simulink model "TSMC_MPC_PMSM"  (R2016b)
settings: Solver=ode23tb  StartTime=0.0  StopTime=0.6  RelTol=1e-4
InitFcn:
  | Ts=10e-6;
  | Rs=0.958;
  | Rf=0.2;
  | Lf=0.002;
  | Cf=0.000021;
  | L=0.000395;
  | Pn=4;
  | flux=0.1827;
  | frq=50;
  | Ld=0.000395;
  | Lq=0.000395;
  | R=0.958;
undefined symbols (not defined in the file or in its folder): DiscIntNeverNeededParam
libraries: powerlib x56, powerlib_extras x2
settings Model: Creator=ChenNingke  LastModifiedBy=CNK
settings SolverCC: MaxConsecutiveZCs=100000  ZeroCrossAlgorithm=Adaptive
settings DebuggingCC: MaskedZcDiagnostic=none

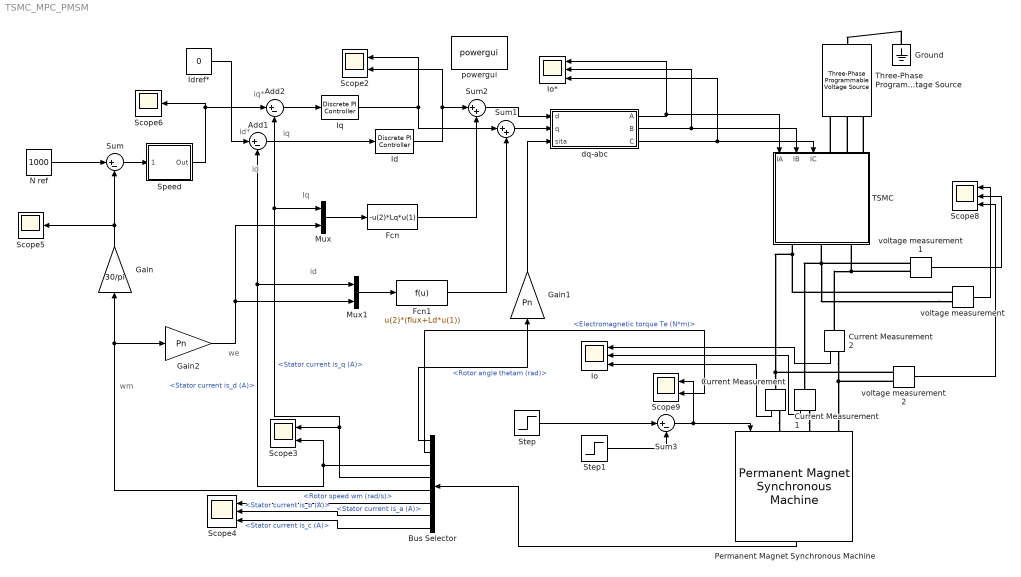
== system TSMC_MPC_PMSM ==
  note: we
  note: wm
  note: iq
  note: id
  note: id*
  note: iq*
  note: id
  note: Iq
  Add1 : Sum  Inputs=|+-
  Add2 : Sum  Inputs=|+-
  Bus Selector : BusSelector  OutputSignals=Rotor angle thetam (rad),Electromagnetic torque Te (N*m),Stator current is_d (A),Stator current is_q (A),Rotor speed wm (rad/s),Stator current is_a (A),Stator current is_b (A),Stator current is_c (A)
  Current Measurement : powerlib/Measurements/Current Measurement  PhasorSimulation=off  OutputType=Complex  PSBequivalent=0
  Current Measurement1 : powerlib/Measurements/Current Measurement  PhasorSimulation=off  OutputType=Complex  PSBequivalent=0
  Current Measurement2 : powerlib/Measurements/Current Measurement  PhasorSimulation=off  OutputType=Complex  PSBequivalent=0
  Fcn : Fcn  Expr=-u(2)*Lq*u(1)
  Fcn1 : Fcn  Expr=u(2)*(flux+Ld*u(1))
  Gain : Gain  Gain=30/pi
  Gain1 : Gain  Gain=Pn
  Gain2 : Gain  Gain=Pn
  Ground : powerlib/Elements/Ground  LConnTagsString=a
  Id : powerlib_extras/Discrete  Control Blocks/Discrete PI Controller  Kp=Ld*1100  Ki=R*1100  Par_Limits=[311*0.9*sqrt(1/3) -311*0.9*sqrt(1/3)]  Init=0  Ts=Ts
  Idref* : Constant  Value=0
  Io : Scope  NumInputPorts=3
  Io* : Scope  NumInputPorts=3
  Iq : powerlib_extras/Discrete  Control Blocks/Discrete PI Controller  Kp=Lq*1100  Ki=R*1100  Par_Limits=[311*0.9*sqrt(1/3) -311*0.9*sqrt(1/3)]  Init=0  Ts=Ts
  Mux : Mux  Inputs=2
  Mux1 : Mux  Inputs=2
  "N ref " : Constant  Value=1000
  Permanent Magnet Synchronous Machine : powerlib/Machines/Permanent Magnet Synchronous Machine  NbPhases=3  FluxDistribution=Sinusoidal  RotorType=Round  MechanicalLoad=Torque Tm  PresetModel=No  ShowDetailedParameters=on  MeasurementBus=off  Resistance=0.958  Inductance=8.5e-3  dqInductances=[Ld,Lq]  La=0.000395  MachineConstant=Flux linkage established by magnets (V.s)  Flux=0.1827  VoltageCst=132.5525  TorqueCst=1.0962  Flat=120  Mechanical=[0.003 0 4 0]  PolePairs=4  InitialConditions=[0,0, 0,0]  InitialConditions5ph=[0 0 0 0 0 0]  TsPowergui=0  TsBlock=-1  RefAngle=90 degrees behind phase A axis (modified Park)
  Scope2 : Scope  NumInputPorts=2
  Scope3 : Scope  NumInputPorts=2
  Scope4 : Scope  NumInputPorts=3
  Scope5 : Scope
  Scope6 : Scope
  Scope8 : Scope  NumInputPorts=3
  Scope9 : Scope  NumInputPorts=2
  Speed : Subsystem  AncestorBlock=|  DialogController=POWERSYS.PowerSysDialog  mask(Discrete PI Controller){Kpw=0.14, Kiw=0.14*50, Ba=0.013, Par_Limits=[15 -15], Init=0, Ts=Ts}
      | powerlib_extras/Discrete 
      | Control Blocks/Discrete
      | PI Controller
      mask prompts: Kpw "Proportional gain (Kp):"; Kiw "Integral gain (Ki):"; Ba "feedback gain (Ba)"; Par_Limits "Output limits: [ Upper   Lower ]"; Init "Output initial value:"; Ts "Sample time:"
      mask help: This block implements a discrete PI controller.
      mask init:
      | UpperLimit=Par_Limits(1);
      | LowerLimit=Par_Limits(2);
      | power_initmask();
      mask Help: This block is part of a subset of blocks in the Extras library that does not have documentation associated with it, other than the block mask description.
      mask Display: disp('PI');
  Step : Step  Time=0.2  After=10  SampleTime=Ts
  Step1 : Step  Time=0.4  After=3  SampleTime=Ts
  Sum : Sum  Inputs=|+-
  Sum1 : Sum  Inputs=|++
  Sum2 : Sum  Inputs=|++
  Sum3 : Sum  Inputs=|+-
  TSMC : Subsystem
  Three-Phase Programmable Voltage Source : powerlib/Electrical Sources/Three-Phase Programmable Voltage Source  PositiveSequence=[220 0 60]  VariationEntity=None  VariationType=Table of time-amplitude pairs  VariationTypeAlt=Step  VariationStep=0.5  VariationRate=10  VariationMagnitude=0.3  VariationFrequency=2  VariationTiming=[1 2]  VariationPhaseA=off  Amplitudes=[1 0.8 1.2 1.0]  TimeValues=[0 0.1 0.15 0.2]  HarmonicGeneration=off  HarmonicA=[3 0.2 -25 0]  HarmonicB=[2 0.15 35 2]  Timing="[0.05  3]"  BusType=swing  Pref=0  Qref=0  Qmin=-inf  Qmax=inf
  dq-abc : Subsystem
  powergui : powerlib/powergui  Priority=1  SimulationMode=Continuous  SolverType=Tustin/Backward Euler (TBE)  SampleTime=50e-6  frequency=60  SPID=off  DisableSnubberDevices=off  DisableRonSwitches=off  DisableVfSwitches=off  SwTol=0  DisplayEquations=off  Interpol=off  ExternalGateDelay=off  methode=off  Ts=10  FunctionMessages=off  echomessages=off  HookPort=off  EnableUseOfTLC=off  x0status=blocks  frequencyindice=0  Pbase=100e6  ErrMax=1e-4  Iterations=50  UnitsV=kV  UnitsW=MW  buscounter=0  RestoreLinks=warning  ResistiveCurrentMeasurement=off  Frange=[0:2:500]  Ylog=off  Xlog=on  ShowGrid=off  save=off  variable=ZData  structure=Io  ZoomFFT=off  StartTime=0.0  cycles=1  DisplayStyle=1  fundamental=60  FreqAxis=off  MaxFrequency=1000  frequencyindicesteady=1  RmsSteady=1  display=off
  voltage measurement : powerlib/Measurements/Voltage Measurement  PhasorSimulation=off  OutputType=Complex  PSBequivalent=0
  voltage measurement1 : powerlib/Measurements/Voltage Measurement  PhasorSimulation=off  OutputType=Complex  PSBequivalent=0
  voltage measurement2 : powerlib/Measurements/Voltage Measurement  PhasorSimulation=off  OutputType=Complex  PSBequivalent=0
  wires:
  dq-abc/1("A ") -> TSMC/1(IA), Io*/1
  dq-abc/2("B ") -> TSMC/2(IB), Io*/2
  Permanent Magnet Synchronous Machine/1 -> Bus Selector/1
  Bus Selector/5 -> Gain2/1, Gain/1  "<Rotor speed wm (rad/s)>"
  "N ref "/1 -> Sum/1
  Speed/1(Out) -> Add2/1, Scope6/1
  Id/1 -> Scope2/2, Sum2/1
  Iq/1 -> Sum1/1, Scope2/1
  Idref*/1 -> Add1/1
  Bus Selector/3 -> Mux1/1, Add1/2, Scope3/2  "<Stator current is_d (A)>"
  Bus Selector/4 -> Scope3/1, Mux/1, Add2/2  "<Stator current is_q (A)>"
  dq-abc/3("C ") -> TSMC/3(IC), Io*/3
  Gain/1 -> Sum/2, Scope5/1
  Bus Selector/8 -> Scope4/3  "<Stator current is_c (A)>"
  Bus Selector/7 -> Scope4/2  "<Stator current is_b (A)>"
  Bus Selector/6 -> Scope4/1  "<Stator current is_a (A)>"
  Bus Selector/1 -> Gain1/1  "<Rotor angle thetam (rad)>"
  Sum/1 -> Speed/1(Error)
  Add2/1 -> Iq/1
  Add1/1 -> Id/1
  Sum2/1 -> dq-abc/1(d)
  Sum1/1 -> dq-abc/2(q)
  voltage measurement/1 -> Scope8/1
  voltage measurement1/1 -> Scope8/2
  voltage measurement2/1 -> Scope8/3
  Current Measurement/1 -> Io/3
  Current Measurement1/1 -> Io/2
  Current Measurement2/1 -> Io/1
  Gain1/1 -> dq-abc/3(sita)
  Mux/1 -> Fcn/1
  Mux1/1 -> Fcn1/1
  Gain2/1 -> Mux/2, Mux1/2
  Fcn/1 -> Sum2/2
  Fcn1/1 -> Sum1/2
  Step/1 -> Sum3/1
  Sum3/1 -> Permanent Magnet Synchronous Machine/1, Scope9/1
  Step1/1 -> Sum3/2
  Bus Selector/2 -> Scope9/2  "<Electromagnetic torque Te (N*m)>"
  connections:
  Current Measurement/LConn1 -- voltage measurement/LConn1 -- TSMC/RConn1 -- voltage measurement2/LConn1
  voltage measurement/LConn2 -- Current Measurement1/LConn1 -- TSMC/RConn2 -- voltage measurement1/LConn1
  Permanent Magnet Synchronous Machine/LConn3 -- Current Measurement2/RConn1 -- voltage measurement2/LConn2
  voltage measurement1/LConn2 -- Current Measurement2/LConn1 -- TSMC/RConn3
  TSMC/LConn3 -- Three-Phase Programmable Voltage Source/RConn3
  TSMC/LConn2 -- Three-Phase Programmable Voltage Source/RConn2
  Ground/LConn1 -- Three-Phase Programmable Voltage Source/LConn1
  TSMC/LConn1 -- Three-Phase Programmable Voltage Source/RConn1
  Current Measurement1/RConn1 -- Permanent Magnet Synchronous Machine/LConn2
  Current Measurement/RConn1 -- Permanent Magnet Synchronous Machine/LConn1

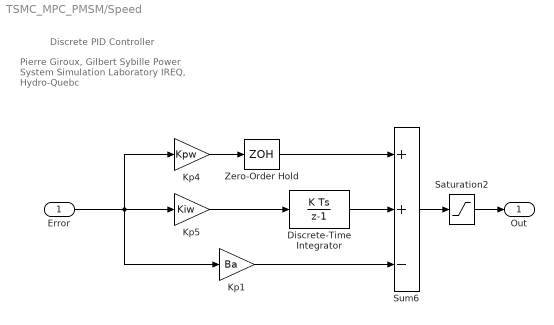
== system TSMC_MPC_PMSM/Speed ==
  note: Discrete PID Controller
  note: Pierre Giroux, Gilbert Sybille
      | Power System Simulation Laboratory
      | IREQ, Hydro-Quebc
  Error : Inport  SampleTime=Ts
  Discrete-Time Integrator : DiscreteIntegrator  InitialCondition=Init  SampleTime=Ts  LimitOutput=on  UpperSaturationLimit=UpperLimit  LowerSaturationLimit=LowerLimit  ICPrevOutput=DiscIntNeverNeededParam  ICPrevScaledInput=DiscIntNeverNeededParam
  Kp1 : Gain  Gain=Ba  SampleTime=Ts  SaturateOnIntegerOverflow=on  OutDataTypeStr=Inherit: Same as input  ParamDataTypeStr=Inherit: Same as input
  Kp4 : Gain  Gain=Kpw  SampleTime=Ts  SaturateOnIntegerOverflow=on  OutDataTypeStr=Inherit: Same as input  ParamDataTypeStr=Inherit: Same as input
  Kp5 : Gain  Gain=Kiw  SampleTime=Ts  SaturateOnIntegerOverflow=on  OutDataTypeStr=Inherit: Same as input  ParamDataTypeStr=Inherit: Same as input
  Saturation2 : Saturate  UpperLimit=UpperLimit  LowerLimit=LowerLimit  SampleTime=Ts
  Sum6 : Sum  Inputs=++-  SampleTime=Ts  SaturateOnIntegerOverflow=on  InputSameDT=on  OutDataTypeStr=Inherit: Same as first input
  Zero-Order Hold : ZeroOrderHold  SampleTime=Ts
  Out : Outport  SampleTime=Ts  InitialOutput=0
  wires:
  Error/1 -> Kp1/1, Kp5/1, Kp4/1
  Zero-Order Hold/1 -> Sum6/1
  Saturation2/1 -> Out/1
  Discrete-Time Integrator/1 -> Sum6/2
  Kp4/1 -> Zero-Order Hold/1
  Kp5/1 -> Discrete-Time Integrator/1
  Sum6/1 -> Saturation2/1
  Kp1/1 -> Sum6/3

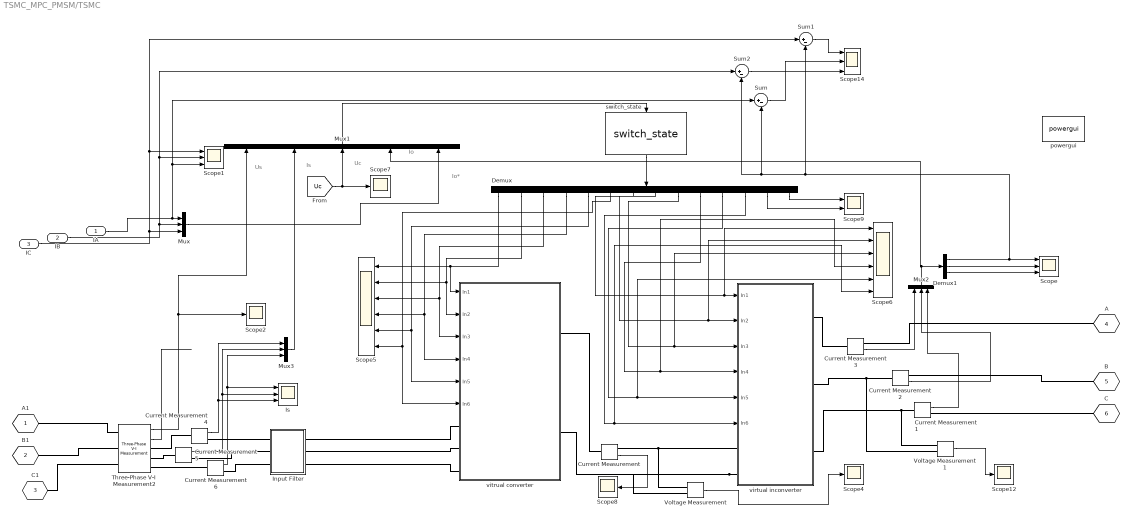
== system TSMC_MPC_PMSM/TSMC ==
  note: Us
  note: Is
  note: Io*
  note: Io
  note: Uc
  IA : Inport
  IB : Inport  Port=2
  IC : Inport  Port=3
  Current Measurement{,1..6} (7 alike) : powerlib/Measurements/Current Measurement  PhasorSimulation=off  OutputType=Complex  PSBequivalent=0
  Demux : Demux  Outputs=14
  Demux1 : Demux  Outputs=3
  Input Filter : Subsystem
  Is : Scope  NumInputPorts=3
  Mux : Mux  Inputs=3
  Mux1 : Mux  Inputs=5
  Mux2 : Mux  Inputs=3
  Mux3 : Mux  Inputs=3
  Scope : Scope  NumInputPorts=3
  Scope1 : Scope  NumInputPorts=3
  Scope{2,4,7..8,12} (5 alike) : Scope
  Scope14 : Scope  NumInputPorts=3
  Scope5 : Scope  NumInputPorts=6
  Scope6 : Scope  NumInputPorts=6
  Scope9 : Scope  NumInputPorts=2
  Sum : Sum  Inputs=|+-
  Sum1 : Sum  Inputs=|+-
  Sum2 : Sum  Inputs=|+-
  Three-Phase V-I Measurement2 : powerlib/Measurements/Three-Phase V-I Measurement  VoltageMeasurement=phase-to-ground  SetLabelV=off  LabelV=Vabc  Vpu=off  VpuLL=off  CurrentMeasurement=yes  SetLabelI=off  LabelI=Iabc  Ipu=off  Pbase=100e6  Vbase=500e3  OutputType=Complex  PhasorSimulation=off  PSBequivalent=0
  Voltage Measurement : powerlib/Measurements/Voltage Measurement  PhasorSimulation=off  OutputType=Complex  PSBequivalent=0
  Voltage Measurement1 : powerlib/Measurements/Voltage Measurement  PhasorSimulation=off  OutputType=Complex  PSBequivalent=0
  powergui : powerlib/powergui  Priority=1  SimulationMode=Continuous  SolverType=Tustin/Backward Euler (TBE)  SampleTime=50e-6  frequency=60  SPID=off  DisableSnubberDevices=off  DisableRonSwitches=off  DisableVfSwitches=off  SwTol=0  DisplayEquations=off  Interpol=off  ExternalGateDelay=off  methode=off  Ts=10  FunctionMessages=off  echomessages=off  HookPort=off  EnableUseOfTLC=off  x0status=blocks  frequencyindice=0  Pbase=100e6  ErrMax=1e-4  Iterations=50  UnitsV=kV  UnitsW=MW  buscounter=0  RestoreLinks=warning  ResistiveCurrentMeasurement=off  Frange=[0:2:500]  Ylog=off  Xlog=on  ShowGrid=off  save=off  variable=ZData  structure=0  ZoomFFT=off  StartTime=0.0  cycles=1  DisplayStyle=1  fundamental=60  FreqAxis=off  MaxFrequency=1000  frequencyindicesteady=1  RmsSteady=1  display=off
  switch_state : S-Function  FunctionName=switch_state  SFunctionDeploymentMode=off  EnableBusSupport=off
  virtual inconverter : Subsystem
  vitrual converter : Subsystem
  A1 : PMIOPort  Tag=PMCPort  Port=1  Side=Left
  B1 : PMIOPort  Tag=PMCPort  Port=2  Side=Left
  C1 : PMIOPort  Tag=PMCPort  Port=3  Side=Left
  A : PMIOPort  Tag=PMCPort  Port=4  Side=Right
  B : PMIOPort  Tag=PMCPort  Port=5  Side=Right
  C : PMIOPort  Tag=PMCPort  Port=6  Side=Right
  wires:
  Three-Phase V-I Measurement2/1 -> Mux1/1, Scope2/1
  Mux3/1 -> Mux1/2
  Mux/1 -> Mux1/5
  Mux2/1 -> Mux1/4, Demux1/1
  switch_state/1 -> Demux/1
  Mux1/1 -> switch_state/1
  Demux/1 -> vitrual converter/1(In1), Scope5/1
  Demux/2 -> vitrual converter/2(In2), Scope5/2
  Demux/3 -> vitrual converter/3(In3), Scope5/3
  Demux/4 -> vitrual converter/4(In4), Scope5/4
  Demux/5 -> vitrual converter/5(In5), Scope5/5
  Demux/6 -> vitrual converter/6(In6), Scope5/6
  Demux/7 -> Scope6/1, virtual inconverter/1(In1)
  Demux/9 -> Scope6/3, virtual inconverter/3(In3)
  Demux/10 -> Scope6/4, virtual inconverter/4(In4)
  Demux/11 -> virtual inconverter/5(In5), Scope6/5
  Demux/12 -> virtual inconverter/6(In6), Scope6/6
  Voltage Measurement/1 -> Scope4/1
  Demux/8 -> Scope6/2, virtual inconverter/2(In2)
  Current Measurement/1 -> Scope8/1
  Demux1/1 -> Sum2/2, Sum/2, Sum1/2, Scope/1
  Demux1/2 -> Scope/2
  Demux1/3 -> Scope/3
  Sum/1 -> Scope14/2
  Sum1/1 -> Scope14/1
  Sum2/1 -> Scope14/3
  Current Measurement1/1 -> Mux2/3
  Current Measurement3/1 -> Mux2/1
  Current Measurement2/1 -> Mux2/2
  Voltage Measurement1/1 -> Scope12/1
  Demux/14 -> Scope9/1
  Demux/13 -> Scope9/2
  Current Measurement4/1 -> Is/3, Mux3/1
  Current Measurement5/1 -> Is/2, Mux3/2
  Current Measurement6/1 -> Is/1, Mux3/3
  [Uc] -> Mux1/3, Scope7/1
  Three-Phase V-I Measurement2/2 -> ?
  IC/1 -> Mux/3, Scope1/1, Sum1/1
  IB/1 -> Mux/2, Scope1/2, Sum2/1
  IA/1 -> Sum/1, Scope1/3, Mux/1
  connections:
  Current Measurement/RConn1 -- Voltage Measurement/LConn1 -- virtual inconverter/LConn1
  virtual inconverter/LConn2 -- vitrual converter/RConn2 -- Voltage Measurement/LConn2
  B/RConn1 -- Current Measurement2/RConn1
  virtual inconverter/RConn3 -- Voltage Measurement1/LConn1 -- Current Measurement1/LConn1
  Current Measurement4/LConn1 -- Three-Phase V-I Measurement2/RConn1
  Current Measurement6/LConn1 -- Three-Phase V-I Measurement2/RConn3
  vitrual converter/RConn1 -- Current Measurement/LConn1
  Current Measurement5/RConn1 -- Input Filter/LConn2
  Three-Phase V-I Measurement2/RConn2 -- Current Measurement5/LConn1
  virtual inconverter/RConn2 -- Voltage Measurement1/LConn2 -- Current Measurement2/LConn1
  vitrual converter/LConn1 -- Input Filter/RConn1
  Input Filter/LConn1 -- Current Measurement4/RConn1
  Current Measurement6/RConn1 -- Input Filter/LConn3
  B1/RConn1 -- Three-Phase V-I Measurement2/LConn2
  vitrual converter/LConn2 -- Input Filter/RConn2
  Input Filter/RConn3 -- vitrual converter/LConn3
  C1/RConn1 -- Three-Phase V-I Measurement2/LConn3
  Current Measurement3/LConn1 -- virtual inconverter/RConn1
  A1/RConn1 -- Three-Phase V-I Measurement2/LConn1
  Current Measurement3/RConn1 -- A/RConn1
  Current Measurement1/RConn1 -- C/RConn1

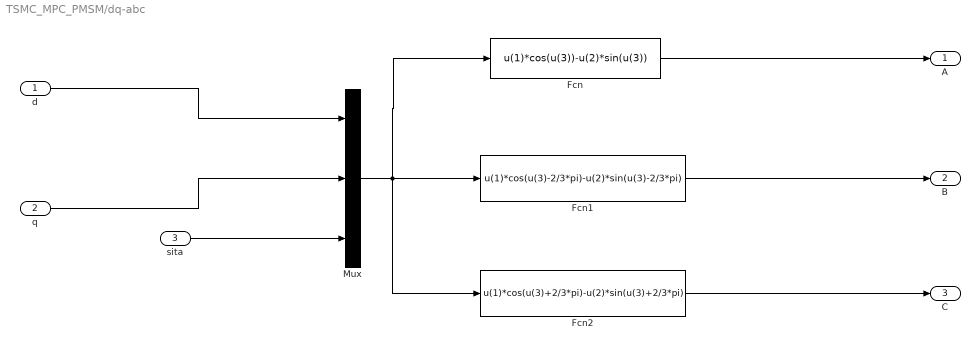
== system TSMC_MPC_PMSM/dq-abc ==
  d : Inport
  q : Inport  Port=2
  sita : Inport  Port=3
  Fcn : Fcn  Expr=u(1)*cos(u(3))-u(2)*sin(u(3))
  Fcn1 : Fcn  Expr=u(1)*cos(u(3)-2/3*pi)-u(2)*sin(u(3)-2/3*pi)
  Fcn2 : Fcn  Expr=u(1)*cos(u(3)+2/3*pi)-u(2)*sin(u(3)+2/3*pi)
  Mux : Mux  Inputs=3
  "A " : Outport
  "B " : Outport  Port=2
  "C " : Outport  Port=3
  wires:
  Fcn/1 -> "A "/1
  Fcn1/1 -> "B "/1
  Mux/1 -> Fcn/1, Fcn1/1, Fcn2/1
  Fcn2/1 -> "C "/1
  sita/1 -> Mux/3
  q/1 -> Mux/2
  d/1 -> Mux/1

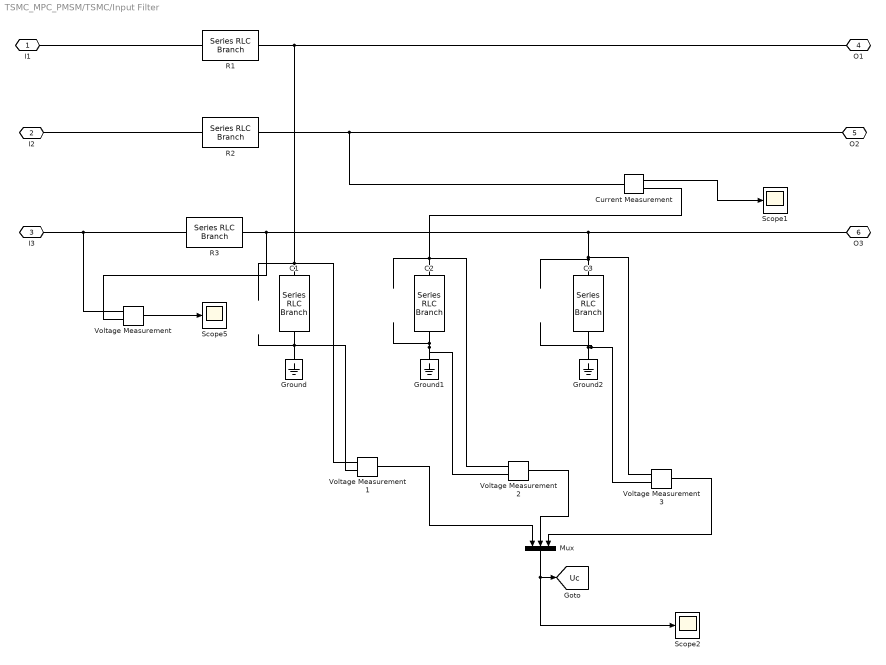
== system TSMC_MPC_PMSM/TSMC/Input Filter ==
  C1 : powerlib/Elements/Series RLC Branch  LConnTagsString=__new0  RConnTagsString=__new0  BranchType=C  Resistance=1  Inductance=1e-3  SetiL0=off  InitialCurrent=0  Capacitance=21e-6  Setx0=off  InitialVoltage=0  Measurements=None
  C2 : powerlib/Elements/Series RLC Branch  LConnTagsString=__new0  RConnTagsString=__new0  BranchType=C  Resistance=1  Inductance=1e-3  SetiL0=off  InitialCurrent=0  Capacitance=21e-6  Setx0=off  InitialVoltage=0  Measurements=None
  C3 : powerlib/Elements/Series RLC Branch  LConnTagsString=__new0  RConnTagsString=__new0  BranchType=C  Resistance=1  Inductance=1e-3  SetiL0=off  InitialCurrent=0  Capacitance=21e-6  Setx0=off  InitialVoltage=0  Measurements=None
  Current Measurement : powerlib/Measurements/Current Measurement  PhasorSimulation=off  OutputType=Complex  PSBequivalent=0
  Ground : powerlib/Elements/Ground  LConnTagsString=a
  Ground1 : powerlib/Elements/Ground  LConnTagsString=a
  Ground2 : powerlib/Elements/Ground  LConnTagsString=a
  Mux : Mux  Inputs=3
  R1 : powerlib/Elements/Series RLC Branch  LConnTagsString=__new0  RConnTagsString=__new0  BranchType=RL  Resistance=0.5  Inductance=0.0004  SetiL0=off  InitialCurrent=0  Capacitance=5e-6  Setx0=off  InitialVoltage=0  Measurements=None
  R2 : powerlib/Elements/Series RLC Branch  LConnTagsString=__new0  RConnTagsString=__new0  BranchType=RL  Resistance=0.5  Inductance=0.0004  SetiL0=off  InitialCurrent=0  Capacitance=5e-6  Setx0=off  InitialVoltage=0  Measurements=None
  R3 : powerlib/Elements/Series RLC Branch  LConnTagsString=__new0  RConnTagsString=__new0  BranchType=RL  Resistance=0.5  Inductance=0.0004  SetiL0=off  InitialCurrent=0  Capacitance=5e-6  Setx0=off  InitialVoltage=0  Measurements=None
  Scope1 : Scope
  Scope2 : Scope
  Scope5 : Scope
  Voltage Measurement{,1..3} (4 alike) : powerlib/Measurements/Voltage Measurement  PhasorSimulation=off  OutputType=Complex  PSBequivalent=0
  I1 : PMIOPort  Port=1  Side=Left
  I2 : PMIOPort  Port=2  Side=Left
  I3 : PMIOPort  Port=3  Side=Left
  O1 : PMIOPort  Port=4  Side=Right
  O2 : PMIOPort  Port=5  Side=Right
  O3 : PMIOPort  Port=6  Side=Right
  tag scope: Uc=global
  wires:
  Voltage Measurement/1 -> Scope5/1
  Current Measurement/1 -> Scope1/1
  Voltage Measurement3/1 -> Mux/3
  Voltage Measurement2/1 -> Mux/2
  Voltage Measurement1/1 -> Mux/1
  Mux/1 -> Scope2/1, [Uc]
  connections:
  Voltage Measurement/LConn2 -- R3/RConn1 -- C3/LConn1 -- Voltage Measurement3/LConn1 -- O3/RConn1
  O2/RConn1 -- R2/RConn1 -- Current Measurement/LConn1
  C1/LConn1 -- Voltage Measurement1/LConn1 -- R1/RConn1 -- O1/RConn1
  C2/LConn1 -- Current Measurement/RConn1 -- Voltage Measurement2/LConn1
  I2/RConn1 -- R2/LConn1
  I1/RConn1 -- R1/LConn1
  I3/RConn1 -- R3/LConn1 -- Voltage Measurement/LConn1
  Ground/LConn1 -- Voltage Measurement1/LConn2 -- C1/RConn1
  Ground1/LConn1 -- Voltage Measurement2/LConn2 -- C2/RConn1
  Ground2/LConn1 -- Voltage Measurement3/LConn2 -- C3/RConn1

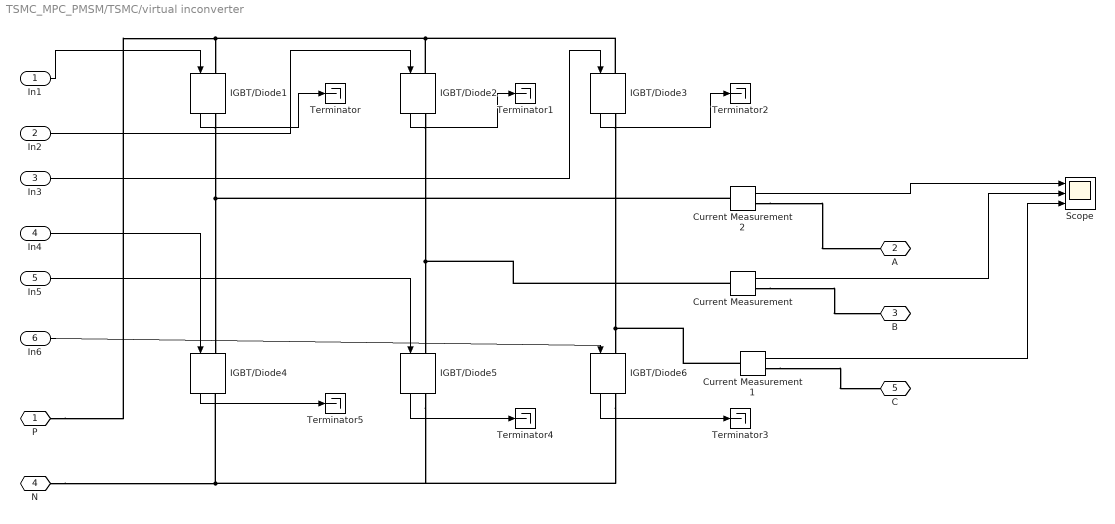
== system TSMC_MPC_PMSM/TSMC/virtual inconverter ==
  In1 : Inport
  In2 : Inport  Port=2
  In3 : Inport  Port=3
  In4 : Inport  Port=4
  In5 : Inport  Port=5
  In6 : Inport  Port=6
  Current Measurement : powerlib/Measurements/Current Measurement  PhasorSimulation=off  OutputType=Complex  PSBequivalent=0
  Current Measurement1 : powerlib/Measurements/Current Measurement  PhasorSimulation=off  OutputType=Complex  PSBequivalent=0
  Current Measurement2 : powerlib/Measurements/Current Measurement  PhasorSimulation=off  OutputType=Complex  PSBequivalent=0
  IGBT/Diode{1..6} (6 alike) : powerlib/Power Electronics/IGBT//Diode  Ron=1e-3  Rs=1e5  Cs=inf  Measurements=on
  Scope : Scope  NumInputPorts=3
  Terminator{,1..5} (6 alike) : Terminator
  P : PMIOPort  Port=1  Side=Left
  A : PMIOPort  Port=2  Side=Right
  B : PMIOPort  Port=3  Side=Right
  N : PMIOPort  Port=4  Side=Left
  C : PMIOPort  Port=5  Side=Right
  wires:
  IGBT/Diode1/1 -> Terminator/1
  IGBT/Diode2/1 -> Terminator1/1
  IGBT/Diode3/1 -> Terminator2/1
  IGBT/Diode6/1 -> Terminator3/1
  IGBT/Diode5/1 -> Terminator4/1
  IGBT/Diode4/1 -> Terminator5/1
  In1/1 -> IGBT/Diode1/1
  In2/1 -> IGBT/Diode2/1
  In3/1 -> IGBT/Diode3/1
  In4/1 -> IGBT/Diode4/1
  In5/1 -> IGBT/Diode5/1
  In6/1 -> IGBT/Diode6/1
  Current Measurement2/1 -> Scope/1
  Current Measurement/1 -> Scope/2
  Current Measurement1/1 -> Scope/3
  connections:
  IGBT/Diode3/LConn1 -- IGBT/Diode2/LConn1 -- P/RConn1 -- IGBT/Diode1/LConn1
  N/RConn1 -- IGBT/Diode6/RConn1 -- IGBT/Diode5/RConn1 -- IGBT/Diode4/RConn1
  IGBT/Diode2/RConn1 -- Current Measurement/LConn1 -- IGBT/Diode5/LConn1
  IGBT/Diode3/RConn1 -- Current Measurement1/LConn1 -- IGBT/Diode6/LConn1
  IGBT/Diode1/RConn1 -- Current Measurement2/LConn1 -- IGBT/Diode4/LConn1
  Current Measurement/RConn1 -- B/RConn1
  Current Measurement1/RConn1 -- C/RConn1
  Current Measurement2/RConn1 -- A/RConn1

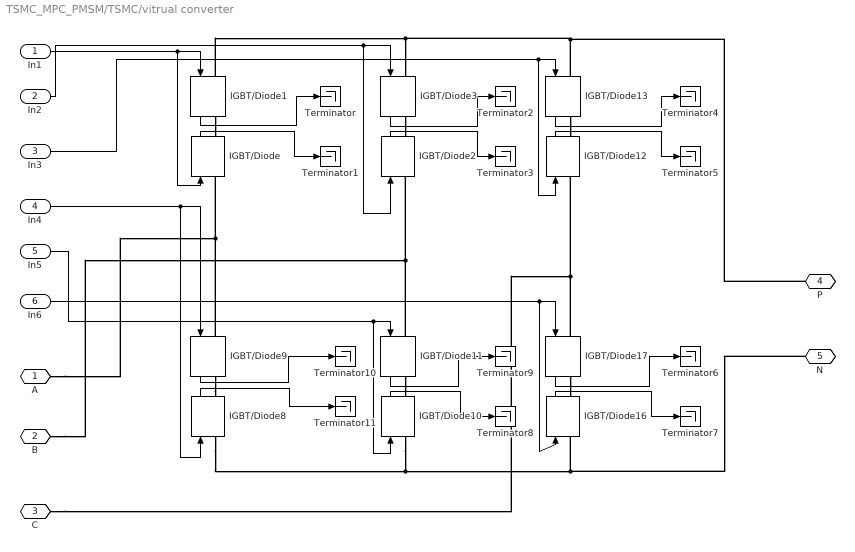
== system TSMC_MPC_PMSM/TSMC/vitrual converter ==
  In1 : Inport
  In2 : Inport  Port=2
  In3 : Inport  Port=3
  In4 : Inport  Port=4
  In5 : Inport  Port=5
  In6 : Inport  Port=6
  IGBT/Diode{,1..3,8..13,16..17} (12 alike) : powerlib/Power Electronics/IGBT//Diode  Ron=1e-3  Rs=1e5  Cs=inf  Measurements=on
  Terminator{,1..11} (12 alike) : Terminator
  A : PMIOPort  Port=1  Side=Left
  B : PMIOPort  Port=2  Side=Left
  C : PMIOPort  Port=3  Side=Left
  P : PMIOPort  Port=4  Side=Right
  N : PMIOPort  Port=5  Side=Right
  wires:
  In1/1 -> IGBT/Diode/1, IGBT/Diode1/1
  IGBT/Diode1/1 -> Terminator/1
  IGBT/Diode/1 -> Terminator1/1
  IGBT/Diode3/1 -> Terminator2/1
  IGBT/Diode2/1 -> Terminator3/1
  IGBT/Diode13/1 -> Terminator4/1
  IGBT/Diode12/1 -> Terminator5/1
  IGBT/Diode17/1 -> Terminator6/1
  IGBT/Diode16/1 -> Terminator7/1
  IGBT/Diode11/1 -> Terminator9/1
  IGBT/Diode10/1 -> Terminator8/1
  IGBT/Diode8/1 -> Terminator11/1
  IGBT/Diode9/1 -> Terminator10/1
  In2/1 -> IGBT/Diode2/1, IGBT/Diode3/1
  In3/1 -> IGBT/Diode12/1, IGBT/Diode13/1
  In4/1 -> IGBT/Diode8/1, IGBT/Diode9/1
  In5/1 -> IGBT/Diode10/1, IGBT/Diode11/1
  In6/1 -> IGBT/Diode16/1, IGBT/Diode17/1
  connections:
  IGBT/Diode1/RConn1 -- IGBT/Diode/RConn1
  IGBT/Diode3/RConn1 -- IGBT/Diode2/RConn1
  IGBT/Diode9/RConn1 -- IGBT/Diode8/RConn1
  IGBT/Diode11/RConn1 -- IGBT/Diode10/RConn1
  IGBT/Diode13/RConn1 -- IGBT/Diode12/RConn1
  IGBT/Diode17/RConn1 -- IGBT/Diode16/RConn1
  IGBT/Diode1/LConn1 -- P/RConn1 -- IGBT/Diode13/LConn1 -- IGBT/Diode3/LConn1
  IGBT/Diode8/LConn1 -- IGBT/Diode16/LConn1 -- N/RConn1 -- IGBT/Diode10/LConn1
  A/RConn1 -- IGBT/Diode9/LConn1 -- IGBT/Diode/LConn1
  IGBT/Diode11/LConn1 -- B/RConn1 -- IGBT/Diode2/LConn1
  IGBT/Diode17/LConn1 -- C/RConn1 -- IGBT/Diode12/LConn1
